simulink model "data_capture_test"  (Simulink 7.0)
settings: Solver=ode45  StartTime=0.0  StopTime=1000  RelTol=1e-3
libraries: xbsIndex_r4 x6, xps_library x4, casper_library x2
settings Model: Creator=sgowda  LastModifiedBy=sgowda

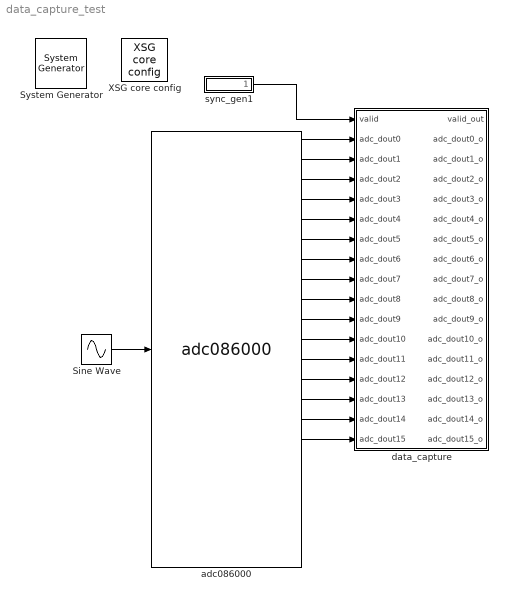
== system data_capture_test ==
  " System Generator" : xbsIndex_r4/ System Generator  Tag=genX  SystemSampleTime=-1  xilinxfamily=virtex5  part=xc5vsx95t  speed=-1  package=ff1136  synthesis_tool=XST  clock_wrapper=Clock Enables  directory=./roach_spec_2adc_borph2/sysgen  testbench=off  simulink_period=1  sysclk_period=10  dcm_input_clock_period=100  incr_netlist=off  trim_vbits=Everywhere in SubSystem  dbl_ovrd=According to Block Masks  core_generation=According to Block Masks  run_coregen=off  deprecated_control=off  eval_field=0  block_type=sysgen
      settings: block_version=10.1.3
  Sine Wave : Sin  Frequency=8*pi/3  Samples=2*pi/4  SampleTime=1/16
  XSG core config : xps_library/XSG core config  Tag=xps:xsg  SystemSampleTime=-1  hw_sys=ROACH:sx95t  ibob_linux=off  clk_src=adc0_clk  iBOB_clk_src=sys_clk  BEE2_ctrl_clk_src=sys_clk  BEE2_usr_clk_src=sys_clk  ROACH_clk_src=adc0_clk  CORR_clk_src=sys_clk  gpio_clk_io_group=iBOB:sma  gpio_clk_bit_index=0  clk_rate=100  sample_period=1  synthesis_tool=XST  mpc_type=powerpc440_ext
  adc086000 : xps_library/adc086000  Tag=xps:adc086000  SystemSampleTime=-1  adc_brd=adc0  adc_clk_rate=400  adc_interleave=on  sample_period=1
  data_capture : Subsystem  AncestorBlock=casper_library/Scopes/data_capture  mask(data_capture){stream_name=adc_dout, nsimult_streams=16}
      mask prompts: stream_name "Stream Name"; nsimult_streams "Number Of Simultaneous Streams"
      mask help:
      | This block is useful for capturing parallel data streams
      | simultaneously and sending the data in structures for analysis
      | using MATLAB.  It is intended as a partial replacement for the
      | Simulink scope block when used with the functions in data_capture_tools.
      |
      | The block does not alter the data at all and costs no hardware
      | because it is purely a simulation block.  The block's Simulink
      | outputs are exactly the same as its inputs with no delay.
      mask init:
      | data_capture_init(gcb, ...
      |     'stream_name', stream_name, ...
      |     'nsimult_streams', nsimult_streams);
  sync_gen1 : Subsystem  mask(sync_gen){sim_acc_len=6, use_soft_reg=off, gen_acc_len=6, fft_size=128, fft_simult_inputs=16, pfb_fir_taps=1, reorder_vec=2, scale=2}
      mask prompts: sim_acc_len "Simulation Accumulation Length"; use_soft_reg "Set on FPGA using software registers"; gen_acc_len "Synthesized Accumulation Length"; fft_size "FFT Size"; fft_simult_inputs "Simultaneous Inputs (FFT)"; pfb_fir_taps "Taps in pfb_fir (use 1 if no pfb_fir)"; reorder_vec "Reorder Orders (e.g. [2 2 2])"
      mask help:
      | sim_acc_len: The accumulation length (i.e. number of spectra to be summed)  that will be used for simulation. If there is no vector accumulator in your design, use 1.  The simulated accumulation length is used to reduce the amount of time the design takes for simulation.
      |
      | gen_acc_len:  The accumaltion length that will be used for generation.
      |
      | fft_size: The size of the FFT.
      |
      | fft_simult_inputs: The number of data inputs into the FFT
      |
      | pfb_fir_taps: The number of PFB filter taps.  IF no pfb_fir in your design, use 1.
      |
      | reorder_vec: A vector of the orders of the reorder blocks inside the FFT.  In your model, the reorder blocks can be found in fft/fft_biplex/biplex_cplx_unscrambler.  The order should be displayed.
      |
      | scale: The amount to scale the sync period by.
      |
      | SyncPeriod=LCM(reorder_vec)*(acc_num)*(pfb_fir_len)*(fft_size/fft_simult_inputs)
      |
      | Check the box if you would like to use a software register
      | to set the runtime sync period.  NOTE THAT THIS RADIO BUTTON RESETS
      | ITSELF SOMETIMES AFTER IT DRAWS THE SOFTWARE REGISTER, CHECK
      | UNDER THE MASK TO VERIFY.
      mask init:
      | sync_gen_init(gcb, ...
      |     'sim_acc_len', sim_acc_len, ...
      |     'fft_size', fft_size, ...
      |     'gen_acc_len', gen_acc_len, ...
      |     'fft_simult_inputs', fft_simult_inputs,...
      |     'pfb_fir_taps', pfb_fir_taps, ...
      |     'reorder_vec', reorder_vec, ...
      |     'use_soft_reg', use_soft_reg, ...
      |     'scale', scale);
      settings: AttributesFormatString=sim_sync_period=96
      mask Help:
      | SyncPeriod=LCM(reorder_vec)*(acc_num)*(pfb_fir_len)*(fft_size/fft_simult_inputs)
      | 
      | See CASPER sync pulse memo for more details.
  wires:
  sync_gen1/1(sync_out) -> data_capture/1(valid)
  adc086000/1 -> data_capture/2(adc_dout0)
  adc086000/2 -> data_capture/3(adc_dout1)
  adc086000/3 -> data_capture/4(adc_dout2)
  adc086000/4 -> data_capture/5(adc_dout3)
  adc086000/5 -> data_capture/6(adc_dout4)
  adc086000/6 -> data_capture/7(adc_dout5)
  adc086000/7 -> data_capture/8(adc_dout6)
  adc086000/8 -> data_capture/9(adc_dout7)
  adc086000/9 -> data_capture/10(adc_dout8)
  adc086000/10 -> data_capture/11(adc_dout9)
  adc086000/11 -> data_capture/12(adc_dout10)
  adc086000/12 -> data_capture/13(adc_dout11)
  adc086000/13 -> data_capture/14(adc_dout12)
  adc086000/14 -> data_capture/15(adc_dout13)
  adc086000/15 -> data_capture/16(adc_dout14)
  adc086000/16 -> data_capture/17(adc_dout15)
  Sine Wave/1 -> adc086000/1

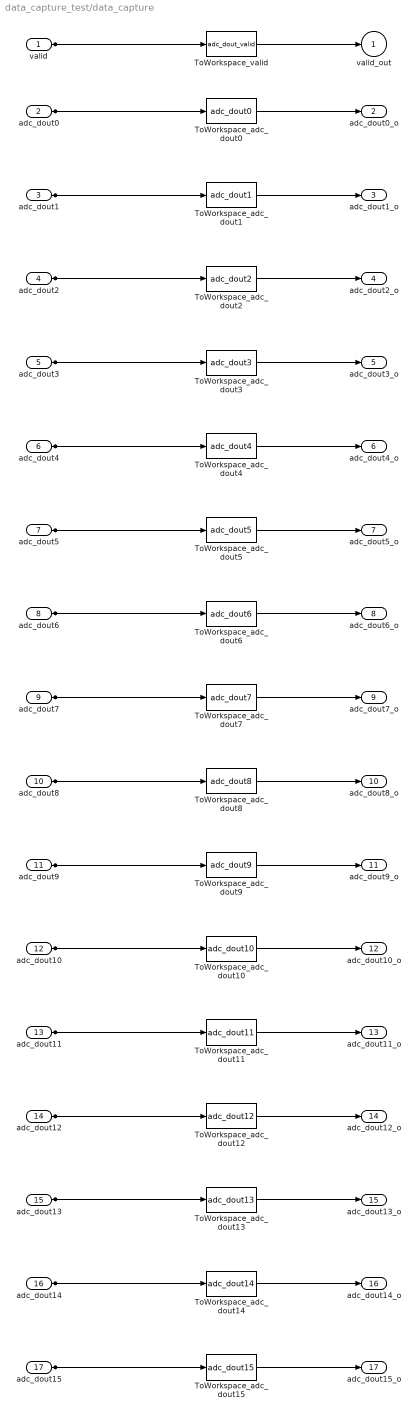
== system data_capture_test/data_capture ==
  valid : Inport  OutDataType=sfix(16)  OutScaling=2^0
  adc_dout0 : Inport  Port=2  OutDataType=sfix(16)  OutScaling=2^0
  adc_dout1 : Inport  Port=3  OutDataType=sfix(16)  OutScaling=2^0
  adc_dout2 : Inport  Port=4  OutDataType=sfix(16)  OutScaling=2^0
  adc_dout3 : Inport  Port=5  OutDataType=sfix(16)  OutScaling=2^0
  adc_dout4 : Inport  Port=6  OutDataType=sfix(16)  OutScaling=2^0
  adc_dout5 : Inport  Port=7  OutDataType=sfix(16)  OutScaling=2^0
  adc_dout6 : Inport  Port=8  OutDataType=sfix(16)  OutScaling=2^0
  adc_dout7 : Inport  Port=9  OutDataType=sfix(16)  OutScaling=2^0
  adc_dout8 : Inport  Port=10  OutDataType=sfix(16)  OutScaling=2^0
  adc_dout9 : Inport  Port=11  OutDataType=sfix(16)  OutScaling=2^0
  adc_dout10 : Inport  Port=12  OutDataType=sfix(16)  OutScaling=2^0
  adc_dout11 : Inport  Port=13  OutDataType=sfix(16)  OutScaling=2^0
  adc_dout12 : Inport  Port=14  OutDataType=sfix(16)  OutScaling=2^0
  adc_dout13 : Inport  Port=15  OutDataType=sfix(16)  OutScaling=2^0
  adc_dout14 : Inport  Port=16  OutDataType=sfix(16)  OutScaling=2^0
  adc_dout15 : Inport  Port=17  OutDataType=sfix(16)  OutScaling=2^0
  ToWorkspace_adc_dout0 : ToWorkspace  VariableName=adc_dout0  SampleTime=-1  SaveFormat=Structure
  ToWorkspace_adc_dout1 : ToWorkspace  VariableName=adc_dout1  SampleTime=-1  SaveFormat=Structure
  ToWorkspace_adc_dout10 : ToWorkspace  VariableName=adc_dout10  SampleTime=-1  SaveFormat=Structure
  ToWorkspace_adc_dout11 : ToWorkspace  VariableName=adc_dout11  SampleTime=-1  SaveFormat=Structure
  ToWorkspace_adc_dout12 : ToWorkspace  VariableName=adc_dout12  SampleTime=-1  SaveFormat=Structure
  ToWorkspace_adc_dout13 : ToWorkspace  VariableName=adc_dout13  SampleTime=-1  SaveFormat=Structure
  ToWorkspace_adc_dout14 : ToWorkspace  VariableName=adc_dout14  SampleTime=-1  SaveFormat=Structure
  ToWorkspace_adc_dout15 : ToWorkspace  VariableName=adc_dout15  SampleTime=-1  SaveFormat=Structure
  ToWorkspace_adc_dout2 : ToWorkspace  VariableName=adc_dout2  SampleTime=-1  SaveFormat=Structure
  ToWorkspace_adc_dout3 : ToWorkspace  VariableName=adc_dout3  SampleTime=-1  SaveFormat=Structure
  ToWorkspace_adc_dout4 : ToWorkspace  VariableName=adc_dout4  SampleTime=-1  SaveFormat=Structure
  ToWorkspace_adc_dout5 : ToWorkspace  VariableName=adc_dout5  SampleTime=-1  SaveFormat=Structure
  ToWorkspace_adc_dout6 : ToWorkspace  VariableName=adc_dout6  SampleTime=-1  SaveFormat=Structure
  ToWorkspace_adc_dout7 : ToWorkspace  VariableName=adc_dout7  SampleTime=-1  SaveFormat=Structure
  ToWorkspace_adc_dout8 : ToWorkspace  VariableName=adc_dout8  SampleTime=-1  SaveFormat=Structure
  ToWorkspace_adc_dout9 : ToWorkspace  VariableName=adc_dout9  SampleTime=-1  SaveFormat=Structure
  ToWorkspace_valid : ToWorkspace  VariableName=adc_dout_valid  SampleTime=-1  SaveFormat=Structure
  valid_out : Outport  OutDataType=sfix(16)  OutScaling=2^0
  adc_dout0_o : Outport  Port=2  OutDataType=sfix(16)  OutScaling=2^0
  adc_dout1_o : Outport  Port=3  OutDataType=sfix(16)  OutScaling=2^0
  adc_dout2_o : Outport  Port=4  OutDataType=sfix(16)  OutScaling=2^0
  adc_dout3_o : Outport  Port=5  OutDataType=sfix(16)  OutScaling=2^0
  adc_dout4_o : Outport  Port=6  OutDataType=sfix(16)  OutScaling=2^0
  adc_dout5_o : Outport  Port=7  OutDataType=sfix(16)  OutScaling=2^0
  adc_dout6_o : Outport  Port=8  OutDataType=sfix(16)  OutScaling=2^0
  adc_dout7_o : Outport  Port=9  OutDataType=sfix(16)  OutScaling=2^0
  adc_dout8_o : Outport  Port=10  OutDataType=sfix(16)  OutScaling=2^0
  adc_dout9_o : Outport  Port=11  OutDataType=sfix(16)  OutScaling=2^0
  adc_dout10_o : Outport  Port=12  OutDataType=sfix(16)  OutScaling=2^0
  adc_dout11_o : Outport  Port=13  OutDataType=sfix(16)  OutScaling=2^0
  adc_dout12_o : Outport  Port=14  OutDataType=sfix(16)  OutScaling=2^0
  adc_dout13_o : Outport  Port=15  OutDataType=sfix(16)  OutScaling=2^0
  adc_dout14_o : Outport  Port=16  OutDataType=sfix(16)  OutScaling=2^0
  adc_dout15_o : Outport  Port=17  OutDataType=sfix(16)  OutScaling=2^0
  wires:
  valid/1 -> ToWorkspace_valid/1, valid_out/1
  adc_dout0/1 -> ToWorkspace_adc_dout0/1, adc_dout0_o/1
  adc_dout1/1 -> ToWorkspace_adc_dout1/1, adc_dout1_o/1
  adc_dout2/1 -> ToWorkspace_adc_dout2/1, adc_dout2_o/1
  adc_dout3/1 -> ToWorkspace_adc_dout3/1, adc_dout3_o/1
  adc_dout4/1 -> ToWorkspace_adc_dout4/1, adc_dout4_o/1
  adc_dout5/1 -> ToWorkspace_adc_dout5/1, adc_dout5_o/1
  adc_dout6/1 -> ToWorkspace_adc_dout6/1, adc_dout6_o/1
  adc_dout7/1 -> ToWorkspace_adc_dout7/1, adc_dout7_o/1
  adc_dout8/1 -> ToWorkspace_adc_dout8/1, adc_dout8_o/1
  adc_dout9/1 -> ToWorkspace_adc_dout9/1, adc_dout9_o/1
  adc_dout10/1 -> ToWorkspace_adc_dout10/1, adc_dout10_o/1
  adc_dout11/1 -> ToWorkspace_adc_dout11/1, adc_dout11_o/1
  adc_dout12/1 -> ToWorkspace_adc_dout12/1, adc_dout12_o/1
  adc_dout13/1 -> ToWorkspace_adc_dout13/1, adc_dout13_o/1
  adc_dout14/1 -> ToWorkspace_adc_dout14/1, adc_dout14_o/1
  adc_dout15/1 -> ToWorkspace_adc_dout15/1, adc_dout15_o/1

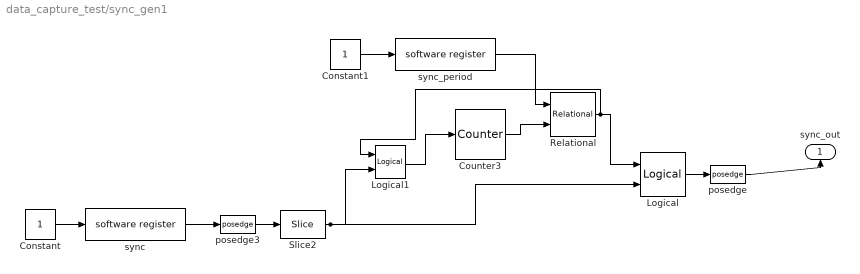
== system data_capture_test/sync_gen1 ==
  Constant : Constant  OutDataType=sfix(16)  OutScaling=2^0
  Constant1 : Constant  OutDataType=sfix(16)  OutScaling=2^0
  Counter3 : xbsIndex_r4/Counter  cnt_type=Free Running  cnt_to=Inf  operation=Up  start_count=0  cnt_by_val=1  arith_type=Unsigned  n_bits=32  bin_pt=0  load_pin=off  rst=on  en=off  explicit_period=off  period=1  dbl_ovrd=off  use_behavioral_HDL=off  use_rpm=on  implementation=Fabric  block_type=counter
      settings: xl_area=[0, 0, 0, 0, 0, 0, 0]
  Logical : xbsIndex_r4/Logical  logical_function=OR  inputs=2  en=off  latency=0  precision=Full  arith_type=Unsigned  n_bits=8  bin_pt=2  align_bp=on  dbl_ovrd=off  block_type=logical
      settings: xl_area=[0, 0, 0, 0, 0, 0, 0]
  Logical1 : xbsIndex_r4/Logical  logical_function=OR  inputs=2  en=off  latency=0  precision=Full  arith_type=Unsigned  n_bits=8  bin_pt=2  align_bp=on  dbl_ovrd=off  block_type=logical
      settings: xl_area=[0, 0, 0, 0, 0, 0, 0]
  Relational : xbsIndex_r4/Relational  mode=a=b  en=off  latency=1  dbl_ovrd=off  block_type=relational
      settings: xl_area=[0, 0, 0, 0, 0, 0, 0]  block_version=10.1.3
  Slice2 : xbsIndex_r4/Slice  nbits=1  boolean_output=on  mode=Lower Bit Location + Width  bit1=0  base1=MSB of Input  bit0=0  base0=LSB of Input  dbl_ovrd=off  block_type=slice
      settings: infoedit="Extracts a given range of bits from each input sample and presents it at the output.  The output type is ordinarily unsigned with binary point at zero, but can be Boolean when the slice is one bit wide.<P><P>Hardware notes: In hardware this block costs nothing."  block_version=10.1.3
  posedge : casper_library/Misc/posedge  Tag=Rising Edge Detector  SystemSampleTime=-1
  posedge3 : casper_library/Misc/posedge  Tag=Rising Edge Detector  SystemSampleTime=-1
  sync : xps_library/software register  Tag=xps:sw_reg  SystemSampleTime=-1  io_dir=From Processor  arith_type=Unsigned  bitwidth=32  bin_pt=0  sample_period=1  gw_name=data_capture_test_sync_gen1_sync_user_data_out
      link override data_capture_test_sync_gen1_sync_user_data_out: arith_type=Unsigned  n_bits=32  bin_pt=0  period=1
      link override fft_16in_sync_gen1_sync_user_data_out: arith_type=Unsigned  n_bits=32  bin_pt=0  period=1
      link override fft_32in_test_sync_gen_sync_user_data_out: arith_type=Unsigned  n_bits=32  bin_pt=0  period=1
      link override fft_8in_test_sync_gen_sync_user_data_out: arith_type=Unsigned  n_bits=32  bin_pt=0  period=1
      link override roach_spec_2adc_borph2_sync_gen1_sync_user_data_out: arith_type=Unsigned  n_bits=32  bin_pt=0  period=1
      link override roach_spec_2adc_borph_backend_test_sync_gen_sync_user_data_out: arith_type=Unsigned  n_bits=32  bin_pt=0  period=1
      link override roach_spec_2adc_borph_sync_gen_sync_user_data_out: arith_type=Unsigned  n_bits=32  bin_pt=0  period=1
      link override untitled_sync_gen1_sync_user_data_out: arith_type=Unsigned  n_bits=32  bin_pt=0  period=1
      link override untitled_sync_gen_sync_user_data_out: arith_type=Unsigned  n_bits=32  bin_pt=0  period=1
  sync_period : xps_library/software register  Tag=xps:sw_reg  SystemSampleTime=-1  io_dir=From Processor  arith_type=Unsigned  bitwidth=32  bin_pt=0  sample_period=1  gw_name=data_capture_test_sync_gen1_sync_period_user_data_out
      link override data_capture_test_sync_gen1_sync_period_user_data_out: arith_type=Unsigned  n_bits=32  bin_pt=0  period=1
      link override fft_16in_sync_gen1_sync_period_user_data_out: arith_type=Unsigned  n_bits=32  bin_pt=0  period=1
      link override fft_16in_sync_gen1_sync_user_data_out: arith_type=Unsigned  n_bits=32  bin_pt=0  period=1
      link override fft_32in_test_sync_gen_sync_user_data_out: arith_type=Unsigned  n_bits=32  bin_pt=0  period=1
      link override fft_8in_test_sync_gen_sync_user_data_out: arith_type=Unsigned  n_bits=32  bin_pt=0  period=1
      link override roach_spec_2adc_borph2_sync_gen1_sync_period_user_data_out: arith_type=Unsigned  n_bits=32  bin_pt=0  period=1
      link override roach_spec_2adc_borph_backend_test_sync_gen_sync_user_data_out: arith_type=Unsigned  n_bits=32  bin_pt=0  period=1
      link override roach_spec_2adc_borph_sync_gen_sync_user_data_out: arith_type=Unsigned  n_bits=32  bin_pt=0  period=1
      link override untitled_sync_gen1_sync_user_data_out: arith_type=Unsigned  n_bits=32  bin_pt=0  period=1
      link override untitled_sync_gen_sync_user_data_out: arith_type=Unsigned  n_bits=32  bin_pt=0  period=1
  sync_out : Outport  Orientation=up  OutDataType=sfix(16)  OutScaling=2^0
  wires:
  Constant/1 -> sync/1
  sync/1 -> posedge3/1
  posedge3/1 -> Slice2/1
  Slice2/1 -> Logical1/2, Logical/2
  Logical1/1 -> Counter3/1
  Counter3/1 -> Relational/2
  Relational/1 -> Logical/1, Logical1/1
  Logical/1 -> posedge/1
  posedge/1 -> sync_out/1
  sync_period/1 -> Relational/1
  Constant1/1 -> sync_period/1
